simulink model "Drone_pid"  (R2017b)
settings: Solver=ode2  StartTime=0.0  StopTime=T  FixedStep=Ts  RelTol=1e-3
values from neighbouring files (symbols this model uses):
  kd_phi = 8    [drone_parameters.m]
  kd_si = 8    [drone_parameters.m]
  kd_theta = 8    [drone_parameters.m]
  kd_z = 8    [drone_parameters.m]
  ki_phi = 0.5    [drone_parameters.m]
  ki_si = 0.5    [drone_parameters.m]
  ki_theta = 0.5    [drone_parameters.m]
  ki_z = 0.5    [drone_parameters.m]
  kp_phi = 7    [drone_parameters.m]
  kp_si = 7    [drone_parameters.m]
  kp_theta = 7    [drone_parameters.m]
  kp_z = 7    [drone_parameters.m]
undefined symbols (not defined in the file or in its folder): droneOrientation, droneparam, dronePos, sigbuilder_block
settings Model: Creator=saad  LastModifiedBy=saad

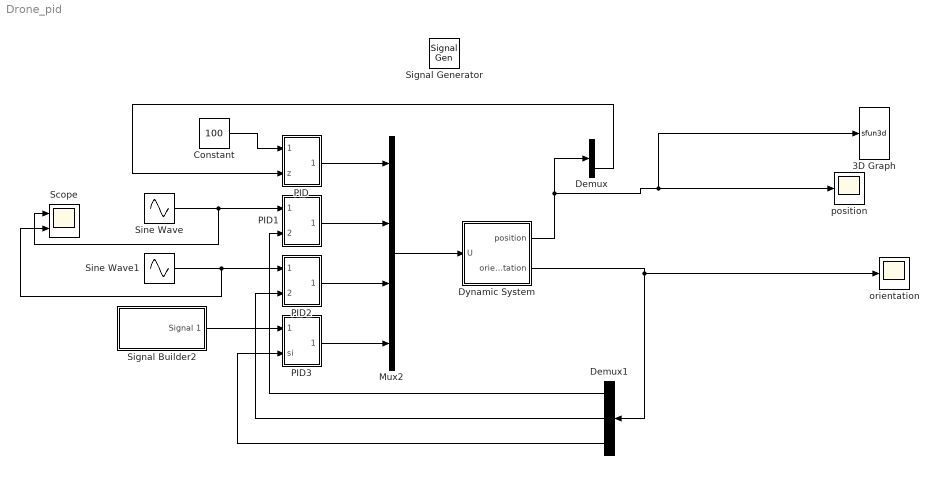
== system Drone_pid ==
  3D Graph : S-Function  LoadFcn=if exist('sfun3d','file'), sfun3d([],[],[],'LoadBlock'); end  FunctionName=sfun3d  Parameters=ax,T,np,cp,gd,ls,mk,mx,hd,tb  SFunctionDeploymentMode=off  EnableBusSupport=off  mask(3D Graph){np=1, ax=[-180 180 -180 180 -180 180], mx=1e10, T=0.002, cp=[-200 -200 200], gd=on, hd=on, tb=off, ls=-, mk=none}
      mask prompts: np "Number of moving points (lines)"; ax "Range: [xmin xmax  ymin ymax zmin zmax]"; mx "Max number of points in each line"; T "Sampling Time"; cp "Camera position (use [0 0 1] for 2D XY view)"; gd "Grid (on|off)"; hd "HeadMarkers (on|off)"; tb "Toolbar (on|off)"; ls "LineStyle"; mk "LineMarker"
      mask help:
      | This block plots the position of several points in the XYZ space. The input contains the coordinates of all the points (x1,y1,z1,x2,y2,z2,...).
      | The number of moving points (lines), the XYZ ranges, sampling time, camera position, and grid (among other things) can be set as mask parameters.
      settings: CopyFcn=if exist('sfun3d','file'), sfun3d([],[],[],'CopyBlock'); end  DeleteFcn=if exist('sfun3d','file'), sfun3d([],[],[],'DeleteBlock'); end  NameChangeFcn=if exist('sfun3d','file'), sfun3d([],[],[],'NameChange'); end
      mask Help:
      | This block plots the position of several points in the XYZ space. The input contains the coordinates of all the points (x1,y1,z1,x2,y2,z2,...).
      | The number of moving points (lines), the XYZ ranges, sampling time, camera position, and grid (among other things) can be set as mask parameters.
      mask TypeOptions ls: - | -- | : | -. | none
      mask TypeOptions mk: none | . | + | o | * | x | square | diamond | v | ^ | > | < | pentagram | hexagram
      mask Display: plot([.05 .95 .95 .05 .05],[.45 .45 .95 .95 .45], 0.5+cos(0:0.1:2*pi)*0.3,0.7+sin(0:0.1:2*pi)*0.2)
  Constant : Constant  Value=100
  Demux : Demux  Outputs=3
  Demux1 : Demux  Outputs=3
  "Dynamic System " : Subsystem
  Mux2 : Mux
  PID : Subsystem
  PID1 : Subsystem
  PID2 : Subsystem
  PID3 : Subsystem
  Scope : Scope  NumInputPorts=2
  Signal Generator : SignalGenerator  Units=rad/sec
  Signal Builder2 : Subsystem  Tag=STV Subsys  LoadFcn=sigbuilder_block('load');  StartFcn=sigbuilder_block('start');  StopFcn=sigbuilder_block('stop');  ClipboardFcn=sigbuilder_block('clipboard');  mask(Sigbuilder block){tuvar=[0:10]}
      mask help: Simulink:masks:SigbuilderBlock_MD
      mask init:
      | if ~strcmp(get_param(bdroot(gcbh),'SimulationStatus'),'stopped') tuvar = sigbuilder_block('maskInit'); end
      settings: CopyFcn=sigbuilder_block('copy');  DeleteFcn=sigbuilder_block('delete');  ModelCloseFcn=sigbuilder_block('modelClose');  PreSaveFcn=sigbuilder_block('preSave');  PauseFcn=sigbuilder_block('pause');  ContinueFcn=sigbuilder_block('continue');  NameChangeFcn=sigbuilder_block('namechange');  OpenFcn=sigbuilder_block('open',[351.75 95.25 550.5 359.25 ]);  CloseFcn=sigbuilder_block('close');
      mask Display: plot(0, 0, 100, 100,[2, 2, 32, 32, 2], [68, 8, 8, 68, 68],[32, 2], [38, 38], [32, 19, 2],[53, 60, 44], [32, 17, 17, 2],[16, 16, 31, 31]);txt = getActiveGroup(gcbh);text(2, 100, txt,'verticalAlignment', 'top');
  Sine Wave : Sin  Frequency=0.2  SampleTime=0
  Sine Wave1 : Sin  Frequency=0.2  Phase=pi/2  SampleTime=0
  orientation : Scope
  "position " : Scope
  wires:
  "Dynamic System "/1("position ") -> Demux/1, 3D Graph/1, "position "/1
  Mux2/1 -> "Dynamic System "/1(U)
  Constant/1 -> PID/1(z_ref)
  Demux/3 -> PID/2(z)
  PID/1(U1) -> Mux2/1
  "Dynamic System "/2(orientation) -> Demux1/1, orientation/1
  Demux1/1 -> PID1/2(phi)
  Demux1/2 -> PID2/2(theta)
  Demux1/3 -> PID3/2(si)
  PID3/1("U4 ") -> Mux2/4
  PID2/1(U3) -> Mux2/3
  PID1/1(U2) -> Mux2/2
  Signal Builder2/1(Signal 1) -> PID3/1(si_ref)
  Sine Wave/1 -> Scope/1, PID1/1(phi_ref)
  Sine Wave1/1 -> Scope/2, PID2/1(theta_ref)

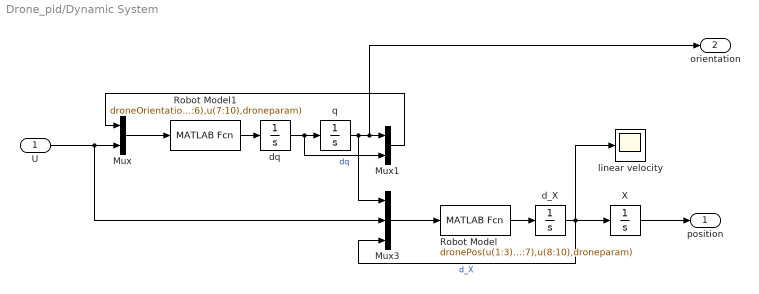
== system Drone_pid/Dynamic System  ==
  U : Inport
  Mux : Mux  Inputs=2
  Mux1 : Mux  Inputs=2
  Mux3 : Mux  Inputs=3
  Robot Model : MATLABFcn  MATLABFcn=dronePos(u(1:3),u(4:7),u(8:10),droneparam)  OutputDimensions=3
  Robot Model1 : MATLABFcn  MATLABFcn=droneOrientation(u(1:3),u(4:6),u(7:10),droneparam)  OutputDimensions=3
  X : Integrator  InitialCondition=droneparam.X0
  d_X : Integrator  InitialCondition=droneparam.X0
  dq : Integrator  InitialCondition=droneparam.q0
  "linear velocity " : Scope
  q : Integrator  InitialCondition=droneparam.q0
  "position " : Outport
  orientation : Outport  Port=2
  wires:
  Mux3/1 -> Robot Model/1
  q/1 -> Mux3/1, orientation/1, Mux1/1
  X/1 -> "position "/1
  U/1 -> Mux3/2, Mux/2
  Mux/1 -> Robot Model1/1
  Mux1/1 -> Mux/1
  dq/1 -> Mux1/2, q/1  "dq"
  Robot Model1/1 -> dq/1
  Robot Model/1 -> d_X/1
  d_X/1 -> "linear velocity "/1, Mux3/3, X/1  "d_X"

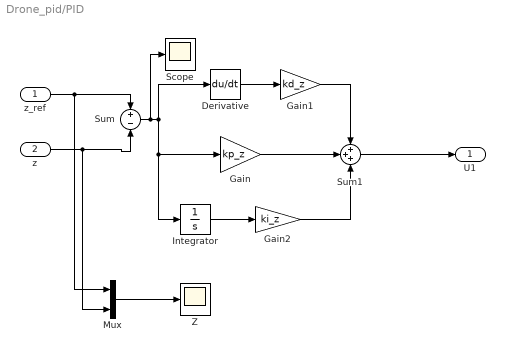
== system Drone_pid/PID ==
  z_ref : Inport
  z : Inport  Port=2
  Derivative : Derivative
  Gain : Gain  Gain=kp_z
  Gain1 : Gain  Gain=kd_z
  Gain2 : Gain  Gain=ki_z
  Integrator : Integrator
  Mux : Mux  Inputs=2
  Scope : Scope
  Sum : Sum  Inputs=+-
  Sum1 : Sum  Inputs=+++
  Z : Scope
  U1 : Outport
  wires:
  Sum/1 -> Gain/1, Integrator/1, Derivative/1, Scope/1
  Integrator/1 -> Gain2/1
  Sum1/1 -> U1/1
  Gain/1 -> Sum1/2
  Gain2/1 -> Sum1/3
  Gain1/1 -> Sum1/1
  Derivative/1 -> Gain1/1
  z/1 -> Mux/2, Sum/2
  z_ref/1 -> Mux/1, Sum/1
  Mux/1 -> Z/1

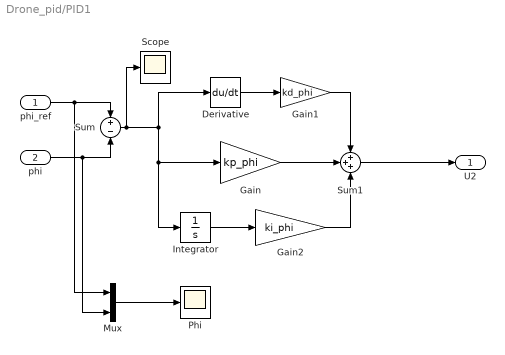
== system Drone_pid/PID1 ==
  phi_ref : Inport
  phi : Inport  Port=2
  Derivative : Derivative
  Gain : Gain  Gain=kp_phi
  Gain1 : Gain  Gain=kd_phi
  Gain2 : Gain  Gain=ki_phi
  Integrator : Integrator
  Mux : Mux  Inputs=2
  Phi : Scope
  Scope : Scope
  Sum : Sum  Inputs=+-
  Sum1 : Sum  Inputs=+++
  U2 : Outport
  wires:
  Derivative/1 -> Gain1/1
  Gain1/1 -> Sum1/1
  phi/1 -> Mux/2, Sum/2
  Gain2/1 -> Sum1/3
  Gain/1 -> Sum1/2
  Sum1/1 -> U2/1
  Integrator/1 -> Gain2/1
  Sum/1 -> Scope/1, Derivative/1, Integrator/1, Gain/1
  phi_ref/1 -> Mux/1, Sum/1
  Mux/1 -> Phi/1

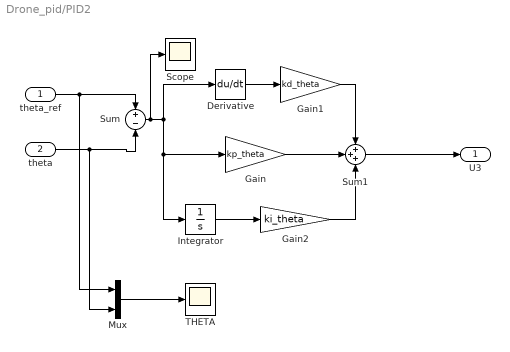
== system Drone_pid/PID2 ==
  theta_ref : Inport
  theta : Inport  Port=2
  Derivative : Derivative
  Gain : Gain  Gain=kp_theta
  Gain1 : Gain  Gain=kd_theta
  Gain2 : Gain  Gain=ki_theta
  Integrator : Integrator
  Mux : Mux  Inputs=2
  Scope : Scope
  Sum : Sum  Inputs=+-
  Sum1 : Sum  Inputs=+++
  "THETA " : Scope
  U3 : Outport
  wires:
  Sum/1 -> Gain/1, Integrator/1, Derivative/1, Scope/1
  Integrator/1 -> Gain2/1
  Sum1/1 -> U3/1
  Gain/1 -> Sum1/2
  Gain2/1 -> Sum1/3
  Gain1/1 -> Sum1/1
  Derivative/1 -> Gain1/1
  theta/1 -> Mux/2, Sum/2
  theta_ref/1 -> Mux/1, Sum/1
  Mux/1 -> "THETA "/1

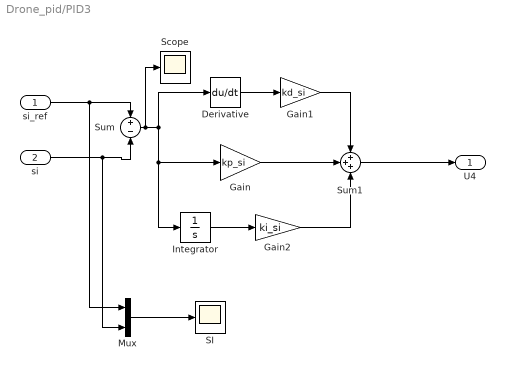
== system Drone_pid/PID3 ==
  si_ref : Inport
  si : Inport  Port=2
  Derivative : Derivative
  Gain : Gain  Gain=kp_si
  Gain1 : Gain  Gain=kd_si
  Gain2 : Gain  Gain=ki_si
  Integrator : Integrator
  Mux : Mux  Inputs=2
  SI : Scope
  Scope : Scope
  Sum : Sum  Inputs=+-
  Sum1 : Sum  Inputs=+++
  "U4 " : Outport
  wires:
  Derivative/1 -> Gain1/1
  Gain1/1 -> Sum1/1
  Gain2/1 -> Sum1/3
  Gain/1 -> Sum1/2
  Sum1/1 -> "U4 "/1
  Integrator/1 -> Gain2/1
  Sum/1 -> Integrator/1, Gain/1, Derivative/1, Scope/1
  si/1 -> Mux/2, Sum/2
  si_ref/1 -> Mux/1, Sum/1
  Mux/1 -> SI/1

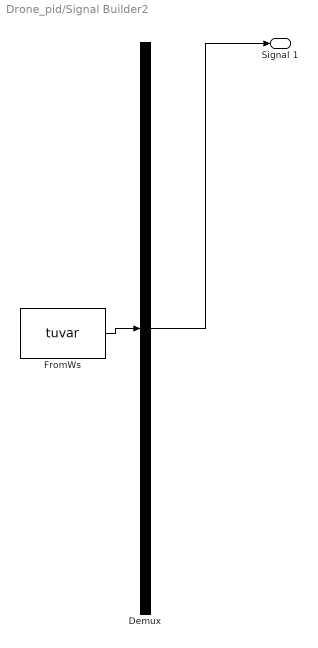
== system Drone_pid/Signal Builder2 ==
  Demux : Demux  Tag=STV Demux  Outputs=1
  FromWs : FromWorkspace  Tag=STV FromWs  VariableName=tuvar  SampleTime=0
      SigBuilderData=|
      | common.afterFinalStr = 'Extrapolate'
      | common.sampleTime = 0
      | dataSet.timeRange = [0 50]
      | dataSet.name = 'Group 1'
      | sbobj.Groups.Name = 'Group 1'
      | sbobj.Groups.Signals.Name = 'Signal 1'
      | sbobj.Groups.Signals.XData = [0 37.2 46.6 50]
      | sbobj.Groups.Signals.YData = [0 -0.0002 -0.0002 -0.0002]
      | sbobj.Groups.TimeRange = [0 50]
  Signal 1 : Outport  Tag=STV Outport
  wires:
  Demux/1 -> Signal 1/1
  FromWs/1 -> Demux/1
